simulink model "sistema"  (R2026a)
settings: Solver=VariableStepAuto
settings Model: Creator=jrcmafc  LastModifiedBy=jrcmafc
settings DataIOCC: TimeSaveName=t
settings DebuggingCC: ArtificialAlgebraicLoopMsg=none  MaxConsecutiveZCsMsg=none

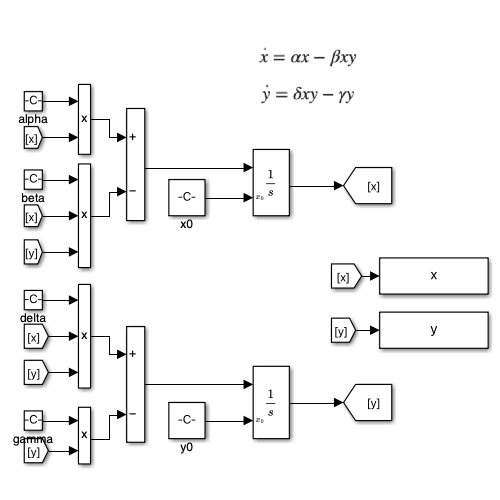
[thumbnail: Simulink's stored preview of the top-level diagram]
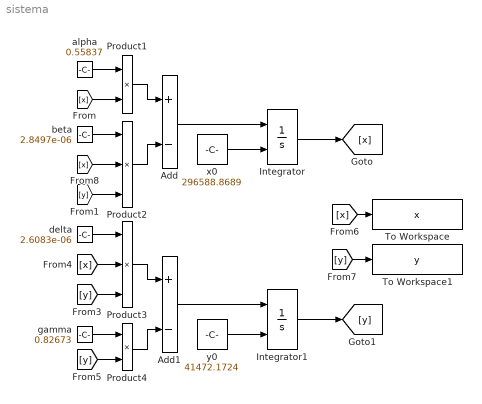
== system sistema ==
  Add : Sum  Inputs=+-
  Add1 : Sum  Inputs=+-
  Integrator : Integrator  InitialConditionSource=external
  Integrator1 : Integrator  InitialConditionSource=external
  Product1 : Product
  Product2 : Product  Inputs=3
  Product3 : Product  Inputs=3
  Product4 : Product
  To Workspace : ToWorkspace  VariableName=x  SampleTime=-1
  To Workspace1 : ToWorkspace  VariableName=y  SampleTime=-1
  alpha : Constant  Value=0.55837
  beta : Constant  Value=2.8497e-06
  delta : Constant  Value=2.6083e-06
  gamma : Constant  Value=0.82673
  x0 : Constant  Value=296588.8689
  y0 : Constant  Value=41472.1724
  wires:
  Add/1 -> Integrator/1
  x0/1 -> Integrator/2
  Add1/1 -> Integrator1/1
  y0/1 -> Integrator1/2
  Integrator/1 -> [x]
  Integrator1/1 -> [y]
  Product1/1 -> Add/1
  Product2/1 -> Add/2
  Product3/1 -> Add1/1
  alpha/1 -> Product1/1
  [x] -> Product1/2
  beta/1 -> Product2/1
  [x] -> Product2/2
  [y] -> Product2/3
  Product4/1 -> Add1/2
  [x] -> Product3/2
  [y] -> Product3/3
  [y] -> Product4/2
  gamma/1 -> Product4/1
  delta/1 -> Product3/1
  [x] -> To Workspace/1
  [y] -> To Workspace1/1
